simulink model "rehastim_gui"  (R2014b)
settings: Solver=FixedStepDiscrete  StartTime=0.0  StopTime=inf  FixedStep=0.01  RelTol=1e-3
undefined symbols (not defined in the file): rehastim_config, sigbuilder_block
libraries: PaPI x1
settings Model: SimulationMode=external  Creator=sven  LastModifiedBy=sven
settings OptimizationCC: OptimizeModelRefInitCode=on  LifeSpan=Inf
settings DebuggingCC: UnderspecifiedInitializationDetection=Classic  MergeDetectMultiDrivingBlocksExec=none  InheritedTsInSrcMsg=none  StateNameClashWarn=warning
settings RTWCC: SystemTargetFile=ert_linux.tlc  MakeCommand="make_rtw OPT_OPTS=\"-DWITH_HW\""  TemplateMakefile=ert_linux.tmf  Description=Linux Embedded Coder  ProcessScript=ert_linux_make_rtw_hook  TargetLang=C++
settings RTWCC: CustomInclude=|
  | /usr/local/MATLAB/R2014b/sys/os/glnxa64/
  | /usr/lib/x86_64-linux-gnu/
  | /usr/include/
settings RTWCC: CustomLibrary=|
  | libstdc++.so.6
  | libgcc_s.so.1
  | libgfortran.so.3
  | libdl.so
  | libboost_system.so
  | libboost_thread.so
  | libboost_signals.so
settings CodeAppCC: IgnoreCustomStorageClasses=off
settings STFCustomTargetCC: TargetLangStandard=C++03 (ISO)  ModelReferenceCompliant=off  CombineOutputUpdateFcns=on  ERTCustomFileBanners=on  SupportContinuousTime=off  SupportNonInlinedSFcns=off  MATLABClassNameForMDSCustomization=Simulink.SoftwareTarget.ERTCustomization  GRTInterface=off  SystemTargetFile=ert_linux.tlc
settings ERTTargetCC: TargetLangStandard=C++03 (ISO)  ModelReferenceCompliant=off  ParMdlRefBuildCompliant=off  CompOptLevelCompliant=off  ConcurrentExecutionCompliant=off  ERTFirstTimeCompliant=off  ModelStepFunctionPrototypeControlCompliant=off  CPPClassGenCompliant=off  ExtMode=on  InlinedParameterPlacement=NonHierarchical  ERTCustomFileTemplate=ert_linux_file_process.tlc

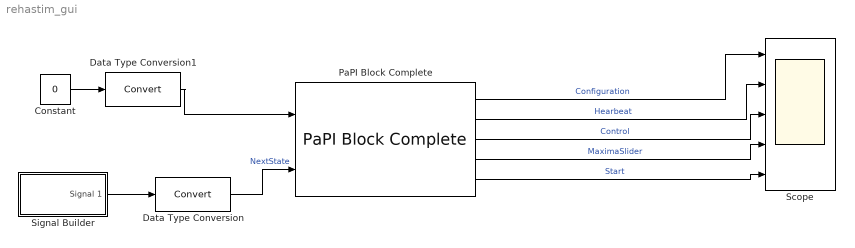
== system rehastim_gui ==
  Constant : Constant  Value=0
  Data Type Conversion : DataTypeConversion
  Data Type Conversion1 : DataTypeConversion
  PaPI Block Complete : PaPI/PaPI Block Complete  amount_parameters=[45,1,1,8,1]  define_inputs=[1]  split_inputs=[1]  json_string=rehastim_config(1)  UDPLocalPort=20001  UDPRemotePort=20000  UDPRemoteIP='127.0.0.1'  output_size=700  sample_time=-1
  Scope : Scope  NumInputPorts=5
      settings: TimeRange=10  YMin=0~1~0~-1~0  YMax=80~2~3~1~1  MaxDataPoints=50000
  Signal Builder : Subsystem  Tag=STV Subsys  LoadFcn=sigbuilder_block('load');  StartFcn=sigbuilder_block('start');  StopFcn=sigbuilder_block('stop');  ClipboardFcn=sigbuilder_block('clipboard');  mask(Sigbuilder block){}
      mask help: Simulink:masks:SigbuilderBlock_MD
      mask init:
      | if ~strcmp(get_param(bdroot(gcbh),'SimulationStatus'),'stopped') tuvar = sigbuilder_block('maskInit'); end
      settings: CopyFcn=sigbuilder_block('copy');  DeleteFcn=sigbuilder_block('delete');  ModelCloseFcn=sigbuilder_block('modelClose');  PreSaveFcn=sigbuilder_block('preSave');  PauseFcn=sigbuilder_block('pause');  ContinueFcn=sigbuilder_block('continue');  NameChangeFcn=sigbuilder_block('namechange');  OpenFcn=sigbuilder_block('open',[437.6 199.2 550.4 400 ]);  CloseFcn=sigbuilder_block('close');
      mask Display: plot(0, 0, 100, 100,[2, 2, 32, 32, 2], [68, 8, 8, 68, 68],[32, 2], [38, 38], [32, 19, 2],[53, 60, 44], [32, 17, 17, 2],[16, 16, 31, 31]);txt = getActiveGroup(gcbh);text(2, 100, txt,'verticalAlignment', 'top');
  wires:
  PaPI Block Complete/1 -> Scope/1  "Configuration"
  PaPI Block Complete/2 -> Scope/2  "Hearbeat"
  PaPI Block Complete/3 -> Scope/3  "Control"
  PaPI Block Complete/4 -> Scope/4  "MaximaSlider"
  Signal Builder/1(Signal 1) -> Data Type Conversion/1
  Data Type Conversion/1 -> PaPI Block Complete/2  "NextState"
  Constant/1 -> Data Type Conversion1/1
  Data Type Conversion1/1 -> PaPI Block Complete/1
  PaPI Block Complete/5 -> Scope/5  "Start"

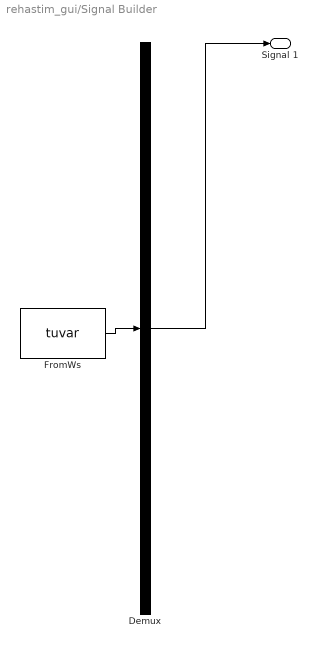
== system rehastim_gui/Signal Builder ==
  Demux : Demux  Tag=STV Demux  Outputs=1
  FromWs : FromWorkspace  Tag=STV FromWs  VariableName=tuvar
      SigBuilderData=|
      | common.afterFinalStr = 'Extrapolate'
      | common.sampleTime = '-1'
      | dataSet.timeRange = [0 40]
      | dataSet.name = 'Group 1'
      | sbobj.Groups.Name = 'Group 1'
      | sbobj.Groups.Signals.Name = 'Signal 1'
      | sbobj.Groups.Signals.XData = [0 14 15 15 17 17 20 20 24 24 27 27 29.3 29.3 35 40]
      | sbobj.Groups.Signals.YData = [1 1 1 2 2 3 3 1 1 2 2 3 3 1 1 1]
      | sbobj.Groups.TimeRange = [0 40]
  Signal 1 : Outport  Tag=STV Outport
  wires:
  Demux/1 -> Signal 1/1
  FromWs/1 -> Demux/1
